simulink model "Rasmusson"  (Simulink 8.8)
settings: Solver=ode15s  StartTime=0.0  StopTime=200  FixedStep=1e-4  MaxStep=0.1  RelTol=1e-6  EnableMultiTasking=on
undefined symbols (not defined in the file): Acap, aKss, ato_f, ato_s, aur, C2, C3, C4, Cai, CaJSR, CaNSR, Cao, Cass, CK1, CK2, Cm, CMDN_tot, CNa1, CNa2, CSQN_tot, ECa_L, ECl, F, GCab, GCaL, GCl_Ca, GKr, GKs, GKss, GKtof, GKtos, GKur, GNa, GNab, HTRPN_tot, HTRPNCa, I1, I1Na, I2, I2Na, I3, ICaL_max, ICNa2, ICNa3, IFNa, IK, iKss, INaK_max, Ip_Ca_max, ito_f, ito_s, iur, ka1, ka2, kb, kb1, kb2, kc1, kc2, kf ... (+45)
(part 2 of 2)

== system Rasmusson/Ionic currents/INa/ONa/CNa1 ==
  note: A44
  Add : Sum  Inputs=+++---
  CNa1 : Constant  Value=CNa1
  Integrator : Integrator  InitialConditionSource=external  InitialCondition=0.279132e-3
  Product{,1..5} (6 alike) : Product  RndMeth=Zero
  tag scope: CNa1=global
  wires:
  [betaNa3] -> Product5/1
  [alphaNa13] -> Product4/1
  [betaNa12] -> Product3/1
  [IFNa] -> Product2/2
  [alphaNa3] -> Product2/1
  [ONa] -> Product1/2
  [betaNa13] -> Product1/1
  [CNa2] -> Product/2
  [alphaNa12] -> Product/1
  Product5/1 -> Add/6
  Product4/1 -> Add/5
  Product3/1 -> Add/4
  Product2/1 -> Add/3
  Product1/1 -> Add/2
  Product/1 -> Add/1
  Add/1 -> Integrator/1
  Integrator/1 -> Product5/2, Product4/2, Product3/2, [CNa1]
  CNa1/1 -> Integrator/2

== system Rasmusson/Ionic currents/INa/ONa/CNa2 ==
  note: A43
  Add : Sum  Inputs=+++---
  CNa2 : Constant  Value=CNa2
  Integrator : Integrator  InitialConditionSource=external  InitialCondition=0.020752
  Product{,1..5} (6 alike) : Product  RndMeth=Zero
  tag scope: CNa2=global
  wires:
  Integrator/1 -> [CNa2], Product3/2, Product4/2, Product5/2
  Add/1 -> Integrator/1
  Product/1 -> Add/1
  Product1/1 -> Add/2
  Product2/1 -> Add/3
  Product3/1 -> Add/4
  Product4/1 -> Add/5
  Product5/1 -> Add/6
  [alphaNa11] -> Product/1
  [CNa3] -> Product/2
  [betaNa12] -> Product1/1
  [CNa1] -> Product1/2
  [alphaNa3] -> Product2/1
  [ICNa2] -> Product2/2
  [betaNa11] -> Product3/1
  [alphaNa12] -> Product4/1
  [betaNa3] -> Product5/1
  CNa2/1 -> Integrator/2

== system Rasmusson/Ionic currents/INa/ONa/CNa3 ==
  note: A42
  Add : Sum  Inputs=+--------
  Constant : Constant
  tag scope: CNa3=global
  wires:
  Add/1 -> [CNa3]
  Constant/1 -> Add/1
  [ONa] -> Add/2
  [CNa1] -> Add/3
  [CNa2] -> Add/4
  [IFNa] -> Add/5
  [I1Na] -> Add/6
  [I2Na] -> Add/7
  [ICNa2] -> Add/8
  [ICNa3] -> Add/9

== system Rasmusson/Ionic currents/INa/ONa/I1Na ==
  note: A47
  Add : Sum  Inputs=++--
  I1Na : Constant  Value=I1Na
  Integrator : Integrator  InitialConditionSource=external  InitialCondition=0.673345e-6
  Product{,1,3,5} (4 alike) : Product  RndMeth=Zero
  tag scope: I1Na=global
  wires:
  Product3/1 -> Add/3
  Product5/1 -> Add/4
  Integrator/1 -> Product5/2, Product3/2, [I1Na]
  Product/1 -> Add/1
  Product1/1 -> Add/2
  [alphaNa5] -> Product5/1
  [betaNa4] -> Product3/1
  [I2Na] -> Product1/2
  [betaNa5] -> Product1/1
  [IFNa] -> Product/2
  [alphaNa4] -> Product/1
  Add/1 -> Integrator/1
  I1Na/1 -> Integrator/2

== system Rasmusson/Ionic currents/INa/ONa/I2Na ==
  note: A48
  Add : Sum  Inputs=+-
  I2Na : Constant  Value=I2Na
  Integrator : Integrator  InitialConditionSource=external  InitialCondition=0.155787e-8
  Product : Product  RndMeth=Zero
  Product5 : Product  RndMeth=Zero
  tag scope: I2Na=global
  wires:
  Add/1 -> Integrator/1
  [alphaNa5] -> Product/1
  [I1Na] -> Product/2
  [betaNa5] -> Product5/1
  Integrator/1 -> [I2Na], Product5/2
  Product5/1 -> Add/2
  Product/1 -> Add/1
  I2Na/1 -> Integrator/2

== system Rasmusson/Ionic currents/INa/ONa/ICNa2 ==
  note: A49
  Add : Sum  Inputs=+++---
  ICNa2 : Constant  Value=ICNa2
  Integrator : Integrator  InitialConditionSource=external  InitialCondition=0.0113879
  Product{,1..5} (6 alike) : Product  RndMeth=Zero
  tag scope: ICNa2=global
  wires:
  [alphaNa3] -> Product5/1
  [alphaNa12] -> Product4/1
  [betaNa11] -> Product3/1
  [CNa2] -> Product2/2
  [betaNa3] -> Product2/1
  [IFNa] -> Product1/2
  [betaNa12] -> Product1/1
  [ICNa3] -> Product/2
  [alphaNa11] -> Product/1
  Product5/1 -> Add/6
  Product4/1 -> Add/5
  Product3/1 -> Add/4
  Product2/1 -> Add/3
  Product1/1 -> Add/2
  Product/1 -> Add/1
  Add/1 -> Integrator/1
  Integrator/1 -> Product5/2, Product4/2, Product3/2, [ICNa2]
  ICNa2/1 -> Integrator/2

== system Rasmusson/Ionic currents/INa/ONa/ICNa3 ==
  note: A50
  Add : Sum  Inputs=++--
  ICNa3 : Constant  Value=ICNa3
  Integrator : Integrator  InitialConditionSource=external  InitialCondition=0.342780
  Product{,1,3,5} (4 alike) : Product  RndMeth=Zero
  tag scope: ICNa3=global
  wires:
  Add/1 -> Integrator/1
  [betaNa11] -> Product/1
  [ICNa2] -> Product/2
  [betaNa3] -> Product1/1
  [CNa3] -> Product1/2
  [alphaNa11] -> Product3/1
  [alphaNa3] -> Product5/1
  Product1/1 -> Add/2
  Product/1 -> Add/1
  Integrator/1 -> [ICNa3], Product3/2, Product5/2
  Product5/1 -> Add/4
  Product3/1 -> Add/3
  ICNa3/1 -> Integrator/2

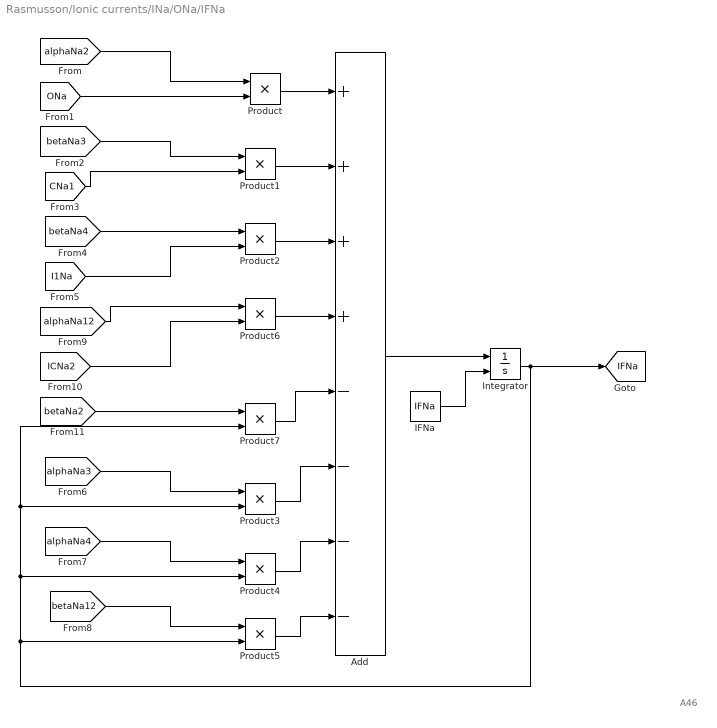
== system Rasmusson/Ionic currents/INa/ONa/IFNa ==
  note: A46
  Add : Sum  Inputs=++++----
  IFNa : Constant  Value=IFNa
  Integrator : Integrator  InitialConditionSource=external  InitialCondition=0.153176e-3
  Product{,1..7} (8 alike) : Product  RndMeth=Zero
  tag scope: IFNa=global
  wires:
  [betaNa12] -> Product5/1
  [alphaNa4] -> Product4/1
  [alphaNa3] -> Product3/1
  [I1Na] -> Product2/2
  [betaNa4] -> Product2/1
  [CNa1] -> Product1/2
  [betaNa3] -> Product1/1
  [ONa] -> Product/2
  [alphaNa2] -> Product/1
  Product2/1 -> Add/3
  Product1/1 -> Add/2
  Product/1 -> Add/1
  Add/1 -> Integrator/1
  Integrator/1 -> Product5/2, Product4/2, Product3/2, Product7/2, [IFNa]
  [ICNa2] -> Product6/2
  [alphaNa12] -> Product6/1
  Product6/1 -> Add/4
  [betaNa2] -> Product7/1
  Product7/1 -> Add/5
  Product3/1 -> Add/6
  Product4/1 -> Add/7
  Product5/1 -> Add/8
  IFNa/1 -> Integrator/2

== system Rasmusson/Ionic currents/INa/ONa/ONa ==
  note: A45
  Add : Sum  Inputs=++--
  Integrator : Integrator  InitialConditionSource=external  InitialCondition=0.713483e-6
  ONa : Constant  Value=ONa
  Product{,1,3,5} (4 alike) : Product  RndMeth=Zero
  tag scope: ONa=global
  wires:
  Add/1 -> Integrator/1
  [alphaNa13] -> Product/1
  [CNa1] -> Product/2
  [betaNa2] -> Product1/1
  [IFNa] -> Product1/2
  [betaNa13] -> Product3/1
  [alphaNa2] -> Product5/1
  Product1/1 -> Add/2
  Product/1 -> Add/1
  Integrator/1 -> [ONa], Product3/2, Product5/2
  Product5/1 -> Add/4
  Product3/1 -> Add/3
  ONa/1 -> Integrator/2

== system Rasmusson/Ionic currents/INa/ONa/alphaNa11 ==
  note: A51
  alphaNa11 : Fcn  Expr=3.802/(0.1027*exp(-(u+2.5)/17)+0.2*exp(-(u+2.5)/150))
  tag scope: alphaNa11=global
  wires:
  [volt] -> alphaNa11/1
  alphaNa11/1 -> [alphaNa11]

== system Rasmusson/Ionic currents/INa/ONa/alphaNa12 ==
  note: A52
  alphaNa12 : Fcn  Expr=3.802/(0.1027*exp(-(u+2.5)/15)+0.23*exp(-(u+2.5)/150))
  tag scope: alphaNa12=global
  wires:
  alphaNa12/1 -> [alphaNa12]
  [volt] -> alphaNa12/1

== system Rasmusson/Ionic currents/INa/ONa/alphaNa13 ==
  note: A53
  alphaNa13 : Fcn  Expr=3.802/(0.1027*exp(-(u+2.5)/12)+0.25*exp(-(u+2.5)/150))
  tag scope: alphaNa13=global
  wires:
  [volt] -> alphaNa13/1
  alphaNa13/1 -> [alphaNa13]

== system Rasmusson/Ionic currents/INa/ONa/alphaNa2 ==
  note: A59
  alphaNa2 : Fcn  Expr=1/(0.188495*exp(-(u+7)/16.6)+0.393956)
  tag scope: alphaNa2=global
  wires:
  alphaNa2/1 -> [alphaNa2]
  [volt] -> alphaNa2/1

== system Rasmusson/Ionic currents/INa/ONa/alphaNa3 ==
  note: A57
  alphaNa3 : Fcn  Expr=7e-7*exp(-(u+7)/7.7)
  tag scope: alphaNa3=global
  wires:
  alphaNa3/1 -> [alphaNa3]
  [volt] -> alphaNa3/1

== system Rasmusson/Ionic currents/INa/ONa/alphaNa4 ==
  note: A61
  Gain : Gain  Gain=0.001
  tag scope: alphaNa4=global
  wires:
  Gain/1 -> [alphaNa4]
  [alphaNa2] -> Gain/1

== system Rasmusson/Ionic currents/INa/ONa/alphaNa5 ==
  note: A63
  Constant : Constant  Value=95000
  Divide : Product  Inputs=*/
  tag scope: alphaNa5=global
  wires:
  Divide/1 -> [alphaNa5]
  [alphaNa2] -> Divide/1
  Constant/1 -> Divide/2

== system Rasmusson/Ionic currents/INa/ONa/betaNa11 ==
  note: A54
  betaNa11 : Fcn  Expr=0.1917*exp(-(u+2.5)/20.3)
  tag scope: betaNa11=global
  wires:
  betaNa11/1 -> [betaNa11]
  [volt] -> betaNa11/1

== system Rasmusson/Ionic currents/INa/ONa/betaNa12 ==
  note: A55
  betaNa12 : Fcn  Expr=0.2*exp(-(u-2.5)/20.3)
  tag scope: betaNa12=global
  wires:
  [volt] -> betaNa12/1
  betaNa12/1 -> [betaNa12]

== system Rasmusson/Ionic currents/INa/ONa/betaNa13 ==
  note: A56
  betaNa13 : Fcn  Expr=0.22*exp(-(u-7.5)/20.3)
  tag scope: betaNa13=global
  wires:
  betaNa13/1 -> [betaNa13]
  [volt] -> betaNa13/1

== system Rasmusson/Ionic currents/INa/ONa/betaNa2 ==
  note: A60
  Divide : Product  Inputs=***//
  tag scope: betaNa2=global
  wires:
  Divide/1 -> [betaNa2]
  [alphaNa13] -> Divide/1
  [alphaNa2] -> Divide/2
  [alphaNa3] -> Divide/3
  [betaNa13] -> Divide/4
  [betaNa3] -> Divide/5

== system Rasmusson/Ionic currents/INa/ONa/betaNa3 ==
  note: A58
  betaNa3 : Fcn  Expr=0.0084+0.00002*(u+7)
  tag scope: betaNa3=global
  wires:
  [volt] -> betaNa3/1
  betaNa3/1 -> [betaNa3]

== system Rasmusson/Ionic currents/INa/ONa/betaNa4 ==
  note: A62
  tag scope: betaNa4=global
  wires:
  [alphaNa3] -> [betaNa4]

== system Rasmusson/Ionic currents/INa/ONa/betaNa5 ==
  note: A64
  Constant : Constant  Value=50
  Divide : Product  Inputs=*/
  tag scope: betaNa5=global
  wires:
  Divide/1 -> [betaNa5]
  [alphaNa3] -> Divide/1
  Constant/1 -> Divide/2

== system Rasmusson/Ionic currents/INaK/fNaK/sigma ==
  note: A110
  Constant : Constant
  Constant1 : Constant  Value=7
  Constant2 : Constant  Value=67300
  Divide : Product  Inputs=*/
  Divide1 : Product  Inputs=*/
  Math Function : Math  SaturateOnIntegerOverflow=on
  Nao : Constant  Value=Nao
  Subtract : Sum  Inputs=+-
  tag scope: sigma=global
  wires:
  Divide/1 -> [sigma]
  Constant1/1 -> Divide/2
  Subtract/1 -> Divide/1
  Constant/1 -> Subtract/2
  Math Function/1 -> Subtract/1
  Nao/1 -> Divide1/1
  Constant2/1 -> Divide1/2
  Divide1/1 -> Math Function/1
